simulink model "ChiefMaster_TTC580"  (R2022b)
settings: Solver=FixedStepAuto  StartTime=0.0  StopTime=10  FixedStep=0.01  RelTol=1e-3
values from neighbouring files (symbols this model uses):
  BattBox1_No = single(1)    [Parameters.m]
  BattBox2_No = single(2)    [Parameters.m]
  BattBox3_No = single(3)    [Parameters.m]
  CurrentLB = single(-3)    [Parameters.m]
  CurrentReductionConstant_Lvl0 = single(0.03)    [Parameters.m]
  CurrentReductionConstant_Lvl1 = single(0.05)    [Parameters.m]
  CurrentReductionConstant_Lvl2 = single(0.07)    [Parameters.m]
  CurrentReductionConstant_Lvl3 = single(0.1)    [Parameters.m]
  CurrentUB = single(3)    [Parameters.m]
  DCHV_Minus_In_Delay_ms = single(500)    [Parameters.m]
  FL_sHVC_CellBalanceVoltage_mV = single(3500)    [Parameters.m]
  FL_sInrushCurrent_dividebyzero = single(0.00001)    [Parameters.m]
  FL_u8HMI_BuzzerTimer = uint8(3)    [Parameters.m]
  IP_boActValue = true    [Parameters.m]
  IP_boDeactValue = false    [Parameters.m]
  IP_boInitValue = false    [Parameters.m]
  IP_s_LB = 18000    [Parameters.m]
  IP_s_UB = 22000    [Parameters.m]
  IP_sBatt1_ChargeCurrentMax_Factor = single(0.1)    [Parameters.m]
  IP_sBatt1_ChargeCurrentMax_LB = single(0)    [Parameters.m]
  IP_sBatt1_ChargeCurrentMax_Offset = single(0)    [Parameters.m]
  IP_sBatt1_ChargeCurrentMax_UB = single(6553.5)    [Parameters.m]
  IP_sBatt1_Current_Factor = single(0.1)    [Parameters.m]
  IP_sBatt1_Current_LB = single(-3276.8)    [Parameters.m]
  IP_sBatt1_Current_Offset = single(0)    [Parameters.m]
  IP_sBatt1_Current_UB = single(3276.8)    [Parameters.m]
  IP_sBatt1_DisChargeCurrentMax_Factor = single(0.1)    [Parameters.m]
  IP_sBatt1_DisChargeCurrentMax_LB = single(0)    [Parameters.m]
  IP_sBatt1_DisChargeCurrentMax_Offset = single(0)    [Parameters.m]
  IP_sBatt1_DisChargeCurrentMax_UB = single(6553.5)    [Parameters.m]
  IP_sBatt1_InsulationResistance_Factor = single(5)    [Parameters.m]
  IP_sBatt1_InsulationResistance_LB = single(0)    [Parameters.m]
  IP_sBatt1_InsulationResistance_Offset = single(0)    [Parameters.m]
  IP_sBatt1_InsulationResistance_UB = single(0)    [Parameters.m]
  IP_sBatt1_LiBa_IntResist_mOhm = single(25)    [Parameters.m]
  IP_sBatt1_SOC_Factor = single(1)    [Parameters.m]
  IP_sBatt1_SOC_LB = single(0)    [Parameters.m]
  IP_sBatt1_SOC_Offset = single(0)    [Parameters.m]
  IP_sBatt1_SOC_UB = single(100)    [Parameters.m]
  IP_sBatt1_SOH_Factor = single(1)    [Parameters.m]
  IP_sBatt1_SOH_LB = single(0)    [Parameters.m]
  IP_sBatt1_SOH_Offset = single(0)    [Parameters.m]
  IP_sBatt1_SOH_UB = single(100)    [Parameters.m]
  IP_sBatt1_Ubatt_Factor = single(0.1)    [Parameters.m]
  IP_sBatt1_Ubatt_LB = single(0)    [Parameters.m]
  IP_sBatt1_Ubatt_Offset = single(0)    [Parameters.m]
  IP_sBatt1_Ubatt_UB = single(6553.5)    [Parameters.m]
  IP_sBatt1_UserRi_Factor = single(1)    [Parameters.m]
  IP_sBatt1_UserRi_LB = single(0)    [Parameters.m]
  IP_sBatt1_UserRi_Offset = single(0)    [Parameters.m]
  IP_sBatt1_UserRi_UB = single(255)    [Parameters.m]
  IP_sBatt1_VoltageAtSensor_Factor = single(0.02)    [Parameters.m]
  IP_sBatt1_VoltageAtSensor_LB = single(0)    [Parameters.m]
  IP_sBatt1_VoltageAtSensor_Offset = single(0)    [Parameters.m]
  IP_sBatt1_VoltageAtSensor_UB = single(1310.7)    [Parameters.m]
  IP_sBatt2_LiBa_IntResist_mOhm = single(25)    [Parameters.m]
  IP_sBatt3_LiBa_IntResist_mOhm = single(25)    [Parameters.m]
  IP_sEM_LB = 2000    [Parameters.m]
  IP_sEM_UB = 8000    [Parameters.m]
  IP_sFB_LB = 5000    [Parameters.m]
  IP_sFB_UB = 10000    [Parameters.m]
  IP_sHVIL_LB = 12000    [Parameters.m]
  IP_sHVIL_UB = 15000    [Parameters.m]
  IP_sLoad_Voltage_Factor = single(1)    [Parameters.m]
  IP_sLoad_Voltage_LB = single(0)    [Parameters.m]
  IP_sLoad_Voltage_Offset = single(0)    [Parameters.m]
  IP_sLoad_Voltage_UB = single(65535)    [Parameters.m]
  IP_u8HVIL_Delay_ms = uint8(100)    [Parameters.m]
  IP_u8HW_IN_delay_ms = uint8(100)    [Parameters.m]
  IT_sInsulationSafeValue_kOhm = single(650)    [Parameters.m]
  IT_u8IMD_DelayTime_s = uint8(20)    [Parameters.m]
  MainHV_Minus_In_Delay = single(5)    [Parameters.m]
  MainHV_StatusDelay = single(5)    [Parameters.m]
  NotAvailable_uint16 = single(65535)    [Parameters.m]
  NotAvailable_uint8 = uint8(255)    [Parameters.m]
  OP_boHVIL_Supply = boolean(1)    [Parameters.m]
  SafeCurrentToCloseHV_A = single(5)    [Parameters.m]
  SafeVoltageToCloseHV_V = single(0.5)    [Parameters.m]
  UnexpectedBattChargingFcn_Available = boolean(1)    [Parameters.m]
  Voltage_NA_UB = uint16(65535)    [Parameters.m]
  VoltageSensorAvailableBB1 = boolean(0)    [Parameters.m]
  VoltageSensorAvailableBB2 = boolean(0)    [Parameters.m]
  VoltageSensorAvailableBB3 = boolean(0)    [Parameters.m]
libraries: simulink x184, Library_DataProcessing_v1_1 x167, Library_DataProcessing_v1 x142, libCM x28
(part 19 of 19)

== stateflow chart ChiefMaster_TTC580/ChiefMaster/Flow Logic/System Status/CurrentPrognosis/BattChargeFcn ==
  state Default
    FL_sST_MaxChargeCurrent = MaxChargeCurrentBatt
    REQ_HV_Open_Batt1 = false
    REQ_HV_Open_Batt2 = false
    REQ_HV_Open_Batt3 = false
    BatteryReadyToShutDown = true
  state RampDown
    FL_sST_MaxChargeCurrent = (FL_sST_MaxChargeCurrent - CurrentReductionConstant)
    REQ_HV_Open_Batt1 = false
    REQ_HV_Open_Batt2 = false
    REQ_HV_Open_Batt3 = false
    BatteryReadyToShutDown = false
  state Stop
    FL_sST_MaxChargeCurrent = 0;
    BatteryReadyToShutDown = true
  state Batt1
    REQ_HV_Open_Batt1 = true
  state Batt2
    REQ_HV_Open_Batt2 = true
  state Batt3
    REQ_HV_Open_Batt3 = true
  (default) -> Default
  RampDown -> Default [order 5] : [Fcn_available == false]
  Default -> RampDown : [ChargeStopPressed == true &&...
      | Fcn_available == true]
  RampDown -> Stop [order 2] : [MaxChargeCurr_fb <= 0]
  RampDown -> Batt1 [order 1] : [HV_ON_Batt1 == 1 &&...
      | Ibatt1 <= CurrentUB]
  Batt1 -> RampDown : [HV_ON_Batt1 == 0 ||...
      | after(20,sec)]
  RampDown -> Batt2 [order 4] : [HV_ON_Batt2 == 1 &&...
      | Ibatt2 <= CurrentUB]
  Batt2 -> RampDown : [HV_ON_Batt2 == 0 ||...
      | after(20,sec)]
  RampDown -> Batt3 [order 3] : [HV_ON_Batt3 == 1 &&...
      | Ibatt3 <= CurrentUB]
  Batt3 -> RampDown : [HV_ON_Batt3 == 0 ||...
      | after(20,sec)]
  data: MaxChargeCurr_fb input; MaxChargeCurrentBatt input; FL_sST_MaxChargeCurrent output; ChargeStopPressed input; HV_ON_Batt1 input; HV_ON_Batt2 input; HV_ON_Batt3 input; Ibatt1 input; Ibatt2 input; Ibatt3 input; REQ_HV_Open_Batt2 output; REQ_HV_Open_Batt3 output; REQ_HV_Open_Batt1 output; Fcn_available input; CurrentReductionConstant input; BatteryReadyToShutDown output; CurrentUB input

== stateflow chart ChiefMaster_TTC580/ChiefMaster/Flow Logic/System Status/EmergencySD/Emergency_Switch_Control/EmergencySwitch_Input_Delay1 ==
  state Initial
    out = IP_boVS_EmergensySwitch;
  state Delay
    out = false;
  state After_delay
    out = IP_boVS_EmergensySwitch;
  (default) -> Initial
  After_delay -> Initial : [IP_boVS_EmergensySwitch == true]
  Initial -> Delay : [IP_boVS_EmergensySwitch == false]
  Delay -> After_delay : [after(10, msec)]
  data: IP_boVS_EmergensySwitch input; out output

== stateflow chart ChiefMaster_TTC580/ChiefMaster/Input Processing/HW Inputs/HVIL/HVIL_Input_Delay ==
  state Initial
    out = HVIL_IN;
  state Delay
    out = true;
  state After_delay
    out = HVIL_IN;
  (default) -> Initial
  After_delay -> Initial : [HVIL_IN == false]
  Initial -> Delay : [HVIL_IN == false]
  Delay -> After_delay : [after(IP_HVIL_Delay_ms, msec)]
  data: HVIL_IN input; out output; IP_HVIL_Delay_ms input

== stateflow chart ChiefMaster_TTC580/ChiefMaster/Input Processing/HW Inputs/HVIL1/HVIL_Input_Delay ==
  state Initial
    out = HVIL_IN;
  state Delay
    out = true;
  state After_delay
    out = HVIL_IN;
  (default) -> Initial
  After_delay -> Initial : [HVIL_IN == false]
  Initial -> Delay : [HVIL_IN == false]
  Delay -> After_delay : [after(IP_HVIL_Delay_ms, msec)]
  data: HVIL_IN input; out output; IP_HVIL_Delay_ms input

== stateflow chart ChiefMaster_TTC580/ChiefMaster/Input Processing/HW Inputs/HVIL2/HVIL_Input_Delay ==
  state Initial
    out = HVIL_IN;
  state Delay
    out = true;
  state After_delay
    out = HVIL_IN;
  (default) -> Initial
  After_delay -> Initial : [HVIL_IN == false]
  Initial -> Delay : [HVIL_IN == false]
  Delay -> After_delay : [after(IP_HVIL_Delay_ms, msec)]
  data: HVIL_IN input; out output; IP_HVIL_Delay_ms input

== stateflow chart ChiefMaster_TTC580/ChiefMaster/Input Translation/Battery Signals/BatteryPackSignals/Subsystem4/IMDOK_Input_Delay ==
  state Initial1
    out = false;
  state After_delay1
    out = In;
  (default) -> Initial1
  Initial1 -> After_delay1 : [after(7,sec)]
  data: out output; In input

== stateflow chart ChiefMaster_TTC580/ChiefMaster/Input Translation/Battery Signals/BatteryPackSignals/Subsystem5/IMDOK_Input_Delay ==
  state Initial1
    out = false;
  state After_delay1
    out = In;
  (default) -> Initial1
  Initial1 -> After_delay1 : [after(7,sec)]
  data: out output; In input

== stateflow chart ChiefMaster_TTC580/ChiefMaster/Input Translation/Battery Signals/BatteryPackSignals/Subsystem6/IMDOK_Input_Delay ==
  state Initial1
    out = false;
  state After_delay1
    out = In;
  (default) -> Initial1
  Initial1 -> After_delay1 : [after(7,sec)]
  data: out output; In input

== stateflow chart ChiefMaster_TTC580/ChiefMaster/Input Translation/Battery Signals/Subsystem7/Subsystem3/IMD_OK ==
  state Default
    IMD_OK=false;
  state Hold3
    IMD_OK=false;
  state Hold
    IMD_OK=true;
  state Hold2
    IMD_OK=true;
  (default) -> Default
  Default -> Hold3 : [IP_boBMS_InsulationReadyOK == true]
  Hold3 -> Hold : [after(IT_u8IMD_DelayTime_s,sec) &&...
      | IP_boBMS_InsulationReadyOK == true]
  (junction 25) -> Default
  Hold -> Hold2 : [Req_IMD == false]
  Hold2 -> (junction 25) : [hasChangedFrom(Req_IMD,false)]
  data: IP_boBMS_InsulationReadyOK input; Req_IMD input; IMD_OK output; IT_u8IMD_DelayTime_s input

== stateflow chart ChiefMaster_TTC580/ChiefMaster/Input Translation/Battery Signals/Subsystem7/Subsystem1/IMD_OK ==
  state Default
    IMD_OK=false;
  state Hold3
    IMD_OK=false;
  state Hold
    IMD_OK=true;
  state Hold2
    IMD_OK=true;
  (default) -> Default
  Default -> Hold3 : [IP_boBMS_InsulationReadyOK == true]
  Hold3 -> Hold : [after(IT_u8IMD_DelayTime_s,sec) &&...
      | IP_boBMS_InsulationReadyOK == true]
  (junction 25) -> Default
  Hold -> Hold2 : [Req_IMD == false]
  Hold2 -> (junction 25) : [hasChangedFrom(Req_IMD,false)]
  data: IP_boBMS_InsulationReadyOK input; Req_IMD input; IMD_OK output; IT_u8IMD_DelayTime_s input

== stateflow chart ChiefMaster_TTC580/ChiefMaster/Input Translation/Battery Signals/Subsystem7/Subsystem2/IMD_OK ==
  state Default
    IMD_OK=false;
  state Hold3
    IMD_OK=false;
  state Hold
    IMD_OK=true;
  state Hold2
    IMD_OK=true;
  (default) -> Default
  Default -> Hold3 : [IP_boBMS_InsulationReadyOK == true]
  Hold3 -> Hold : [after(IT_u8IMD_DelayTime_s,sec) &&...
      | IP_boBMS_InsulationReadyOK == true]
  (junction 25) -> Default
  Hold -> Hold2 : [Req_IMD == false]
  Hold2 -> (junction 25) : [hasChangedFrom(Req_IMD,false)]
  data: IP_boBMS_InsulationReadyOK input; Req_IMD input; IMD_OK output; IT_u8IMD_DelayTime_s input
